simulink model "simlab5"  (R2025b)
settings: Solver=FixedStepAuto  StartTime=0.0  StopTime=10  FixedStep=0.001  RelTol=1e-3
values from neighbouring files (symbols this model uses):
  ld1 = ld1{1}    [lab5.m]
  ld2 = ld2{1}    [lab5.m]
  Lr1 = q01*md1    [lab5.m]
  Lr2 = q02*md2    [lab5.m]
  md1 = md1{1}    [lab5.m]
  md2 = md2{1}    [lab5.m]
  Mr1 = [1 -ld1*q01]    [lab5.m]
  Mr2 = [1 -ld2*q02]    [lab5.m]
  Tp = 0.1    [lab5.m]
undefined symbols (not defined in the file or in its folder): dspblkCoreblockFVToolHelper, gcbh
settings Model: Creator=LabB2s218-04  LastModifiedBy=Maciek
settings RTWCC: GPUComputeCapability=3.5

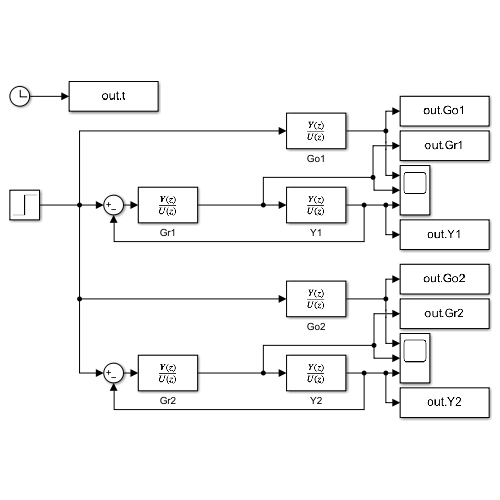
[thumbnail: Simulink's stored preview of the top-level diagram]
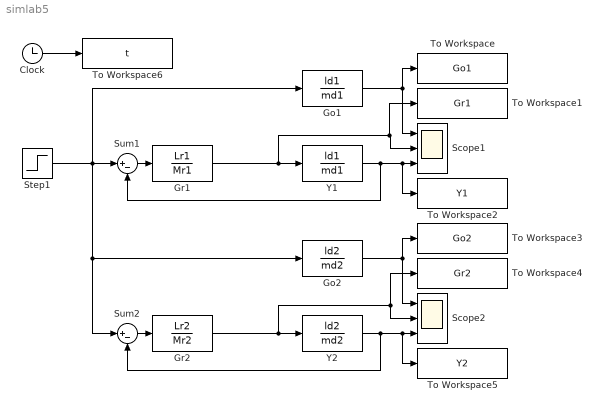
== system simlab5 ==
  Clock : Clock
  Go1 : DiscreteTransferFcn  LoadFcn=dspblkCoreblockFVToolHelper(gcbh,'load');  Numerator=ld1  Denominator=md1  SampleTime=Tp
      settings: CopyFcn=dspblkCoreblockFVToolHelper(gcbh,'copy');  DeleteFcn=dspblkCoreblockFVToolHelper(gcbh,'close');  ModelCloseFcn=dspblkCoreblockFVToolHelper(gcbh,'close');  PreSaveFcn=dspblkCoreblockFVToolHelper(gcbh,'presave');  PostSaveFcn=dspblkCoreblockFVToolHelper(gcbh,'postsave');  CloseFcn=dspblkCoreblockFVToolHelper(gcbh,'close');
  Go2 : DiscreteTransferFcn  LoadFcn=dspblkCoreblockFVToolHelper(gcbh,'load');  Numerator=ld2  Denominator=md2  SampleTime=Tp
      settings: CopyFcn=dspblkCoreblockFVToolHelper(gcbh,'copy');  DeleteFcn=dspblkCoreblockFVToolHelper(gcbh,'close');  ModelCloseFcn=dspblkCoreblockFVToolHelper(gcbh,'close');  PreSaveFcn=dspblkCoreblockFVToolHelper(gcbh,'presave');  PostSaveFcn=dspblkCoreblockFVToolHelper(gcbh,'postsave');  CloseFcn=dspblkCoreblockFVToolHelper(gcbh,'close');
  Gr1 : DiscreteTransferFcn  LoadFcn=dspblkCoreblockFVToolHelper(gcbh,'load');  Numerator=Lr1  Denominator=Mr1  SampleTime=Tp
      settings: CopyFcn=dspblkCoreblockFVToolHelper(gcbh,'copy');  DeleteFcn=dspblkCoreblockFVToolHelper(gcbh,'close');  ModelCloseFcn=dspblkCoreblockFVToolHelper(gcbh,'close');  PreSaveFcn=dspblkCoreblockFVToolHelper(gcbh,'presave');  PostSaveFcn=dspblkCoreblockFVToolHelper(gcbh,'postsave');  CloseFcn=dspblkCoreblockFVToolHelper(gcbh,'close');
  Gr2 : DiscreteTransferFcn  LoadFcn=dspblkCoreblockFVToolHelper(gcbh,'load');  Numerator=Lr2  Denominator=Mr2  SampleTime=Tp
      settings: CopyFcn=dspblkCoreblockFVToolHelper(gcbh,'copy');  DeleteFcn=dspblkCoreblockFVToolHelper(gcbh,'close');  ModelCloseFcn=dspblkCoreblockFVToolHelper(gcbh,'close');  PreSaveFcn=dspblkCoreblockFVToolHelper(gcbh,'presave');  PostSaveFcn=dspblkCoreblockFVToolHelper(gcbh,'postsave');  CloseFcn=dspblkCoreblockFVToolHelper(gcbh,'close');
  Scope1 : Scope  NumInputPorts=3
      settings: ActiveDisplayYMinimum=-1.2610501455438434  ActiveDisplayYMaximum=2.5014902709909865
  Scope2 : Scope  NumInputPorts=3
      settings: ActiveDisplayYMinimum=-22.042622087174827  ActiveDisplayYMaximum=12.926280964667624
  Step1 : Step  Time=0  SampleTime=Tp
  Sum1 : Sum  Inputs=|+-
  Sum2 : Sum  Inputs=|+-
  To Workspace : ToWorkspace  VariableName=Go1  SaveFormat=Timeseries  SampleTime=Tp
  To Workspace1 : ToWorkspace  VariableName=Gr1  SaveFormat=Timeseries  SampleTime=Tp
  To Workspace2 : ToWorkspace  VariableName=Y1  SaveFormat=Timeseries  SampleTime=Tp
  To Workspace3 : ToWorkspace  VariableName=Go2  SaveFormat=Timeseries  SampleTime=Tp
  To Workspace4 : ToWorkspace  VariableName=Gr2  SaveFormat=Timeseries  SampleTime=Tp
  To Workspace5 : ToWorkspace  VariableName=Y2  SaveFormat=Timeseries  SampleTime=Tp
  To Workspace6 : ToWorkspace  VariableName=t  SaveFormat=Timeseries  SampleTime=Tp
  Y1 : DiscreteTransferFcn  LoadFcn=dspblkCoreblockFVToolHelper(gcbh,'load');  Numerator=ld1  Denominator=md1  SampleTime=Tp
      settings: CopyFcn=dspblkCoreblockFVToolHelper(gcbh,'copy');  DeleteFcn=dspblkCoreblockFVToolHelper(gcbh,'close');  ModelCloseFcn=dspblkCoreblockFVToolHelper(gcbh,'close');  PreSaveFcn=dspblkCoreblockFVToolHelper(gcbh,'presave');  PostSaveFcn=dspblkCoreblockFVToolHelper(gcbh,'postsave');  CloseFcn=dspblkCoreblockFVToolHelper(gcbh,'close');
  Y2 : DiscreteTransferFcn  LoadFcn=dspblkCoreblockFVToolHelper(gcbh,'load');  Numerator=ld2  Denominator=md2  SampleTime=Tp
      settings: CopyFcn=dspblkCoreblockFVToolHelper(gcbh,'copy');  DeleteFcn=dspblkCoreblockFVToolHelper(gcbh,'close');  ModelCloseFcn=dspblkCoreblockFVToolHelper(gcbh,'close');  PreSaveFcn=dspblkCoreblockFVToolHelper(gcbh,'presave');  PostSaveFcn=dspblkCoreblockFVToolHelper(gcbh,'postsave');  CloseFcn=dspblkCoreblockFVToolHelper(gcbh,'close');
  wires:
  Sum1/1 -> Gr1/1
  Y1/1 -> Sum1/2, To Workspace2/1, Scope1/3
  Gr1/1 -> To Workspace1/1, Scope1/2, Y1/1
  Go1/1 -> To Workspace/1, Scope1/1
  Y2/1 -> Sum2/2, To Workspace5/1, Scope2/3
  Sum2/1 -> Gr2/1
  Gr2/1 -> To Workspace4/1, Scope2/2, Y2/1
  Step1/1 -> Sum2/1, Go2/1, Go1/1, Sum1/1
  Go2/1 -> Scope2/1, To Workspace3/1
  Clock/1 -> To Workspace6/1
